simulink model "pingtai_with_control_gaijin1PIDNN3_2"  (R2014a)
settings: Solver=ode23t  StartTime=0.0  StopTime=100.0  MaxStep=1e-2  RelTol=1e-3
values from neighbouring files (symbols this model uses):
  m = 0    [cs_search.m]    (also in pso_search.m = n)
  s = new_nest(j,:)    [empty_nests.m]    (also in get_cuckoos.m = s+stepsize.*randn(size(s)); pso_search.m = newnest(i,:); simplebounds.m = ns_tmp)
undefined symbols (not defined in the file or in its folder): mpidnn, sigbuilder_block, WW, X, Y, Z
libraries: fl_lib x68, sm_lib x65, nesl_utility x65, simulink x18, sm_radial_engine_lib x8, sdl_lib x8, elec_lib x4
(part 5 of 5)

== system pingtai_with_control_gaijin1PIDNN3_2/zhitui3/shengjiagnji2/Sensor 1 ==
  Ideal Rotational Motion Sensor : fl_lib/Mechanical/Mechanical Sensors/Ideal Rotational Motion Sensor  offset=0 rad
  MRR3 : fl_lib/Mechanical/Rotational Elements/Mechanical Rotational Reference
  PS-Simulink Converter : nesl_utility/PS-Simulink Converter  PhysicalDomain=network_engine_domain  SubClassName=ps_output  LeftPortType=input  RightPortType=output  PseudoPeriodic=off  Frequencies=[]  Unit=1  AffineConversion=off
  R : PMIOPort  Port=1  Side=Left
  w : Outport
  wires:
  PS-Simulink Converter/1 -> w/1
  connections:
  MRR3/LConn1 -- Ideal Rotational Motion Sensor/RConn1
  Ideal Rotational Motion Sensor/RConn2 -- PS-Simulink Converter/LConn1
  R/RConn1 -- Ideal Rotational Motion Sensor/LConn1

== system pingtai_with_control_gaijin1PIDNN3_2/zhitui4/shengjiagnji2/	ITAE ==
  In1 : Inport
  In2 : Inport  Port=2
  In3 : Inport  Port=3
  Abs : Abs  ZeroCross=off  SaturateOnIntegerOverflow=on
  Add : Sum  Inputs=+-
  Add1 : Sum
  Display : Display
  Display1 : Display
  Gain : Gain  Gain=50
  Gain1 : Gain  Gain=80
  Integrator1 : Integrator
  MinMax Running Resettable : simulink/Math Operations/MinMax Running Resettable  Function=max  vinit=0.0
  Product1 : Product  SaturateOnIntegerOverflow=on  OutDataTypeStr=Inherit: Same as first input
  time : Clock
  Out1 : Outport
  wires:
  Add1/1 -> Out1/1
  Gain1/1 -> Add1/2
  Gain/1 -> Add1/1
  In3/1 -> Add/2
  In2/1 -> Add/1
  MinMax Running Resettable/1 -> Display1/1, Gain1/1
  Add/1 -> MinMax Running Resettable/1
  In1/1 -> Abs/1
  Abs/1 -> Product1/2
  Product1/1 -> Integrator1/1
  Integrator1/1 -> Display/1, Gain/1
  time/1 -> Product1/1

== system pingtai_with_control_gaijin1PIDNN3_2/zhitui4/shengjiagnji2/Sensor 1 ==
  Ideal Rotational Motion Sensor : fl_lib/Mechanical/Mechanical Sensors/Ideal Rotational Motion Sensor  offset=0 rad
  MRR3 : fl_lib/Mechanical/Rotational Elements/Mechanical Rotational Reference
  PS-Simulink Converter : nesl_utility/PS-Simulink Converter  PhysicalDomain=network_engine_domain  SubClassName=ps_output  LeftPortType=input  RightPortType=output  PseudoPeriodic=off  Frequencies=[]  Unit=1  AffineConversion=off
  R : PMIOPort  Port=1  Side=Left
  w : Outport
  wires:
  PS-Simulink Converter/1 -> w/1
  connections:
  R/RConn1 -- Ideal Rotational Motion Sensor/LConn1
  Ideal Rotational Motion Sensor/RConn2 -- PS-Simulink Converter/LConn1
  MRR3/LConn1 -- Ideal Rotational Motion Sensor/RConn1
